simulink model "UseSimDynamicsData"  (R2018b)
settings: configuration reference "RPi_DynamicsRate" (kept outside this file)
values from neighbouring files (symbols this model uses):
  rangeSensorAngBody = [0; 90*dtr; 180*dtr; 270*dtr]    [loadSensorData.m]
  rangeSensorFOV = [0*dtr; 0*dtr; 0*dtr; 0*dtr]    [loadSensorData.m]
  wallBounds = [wallA; wallB; wallC; wallD]    [loadSensorData.m]
undefined symbols (not defined in the file or in its folder): rangeSensorLocBody
settings Model: Creator=barthal  LastModifiedBy=barthal
settings ConfigSetRef: SourceLocation=Base Workspace

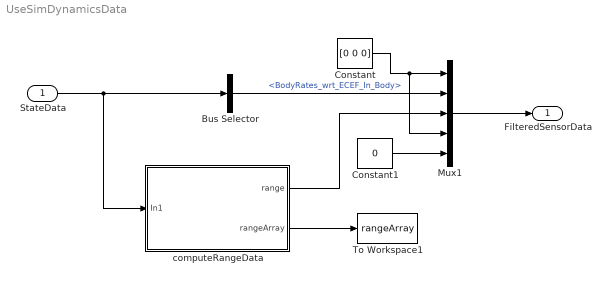
== system UseSimDynamicsData ==
  StateData : Inport  OutDataTypeStr=Bus: FullStateBus
  Bus Selector : BusSelector  OutputSignals=RotState_Body_ECEF.BodyRates_wrt_ECEF_In_Body
  Constant : Constant  Value=[0 0 0]
  Constant1 : Constant  Value=0
  Mux1 : Mux  Inputs=5
  To Workspace1 : ToWorkspace  VariableName=rangeArray  SaveFormat=Timeseries  SampleTime=-1
  computeRangeData : Subsystem
  FilteredSensorData : Outport
  wires:
  StateData/1 -> Bus Selector/1, computeRangeData/1(In1)
  Constant/1 -> Mux1/4, Mux1/1
  Mux1/1 -> FilteredSensorData/1
  computeRangeData/1(range) -> Mux1/3
  computeRangeData/2(rangeArray) -> To Workspace1/1
  Bus Selector/1 -> Mux1/2  "<BodyRates_wrt_ECEF_In_Body>"
  Constant1/1 -> Mux1/5

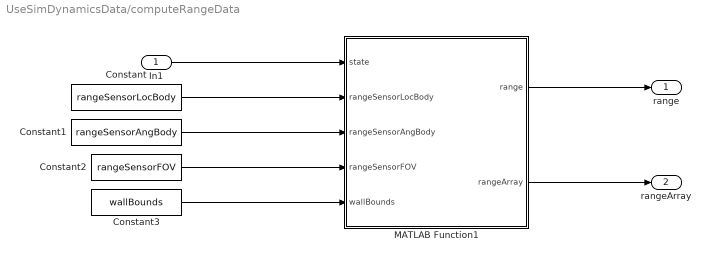
== system UseSimDynamicsData/computeRangeData ==
  In1 : Inport
  Constant : Constant  Value=rangeSensorLocBody
  Constant1 : Constant  Value=rangeSensorAngBody
  Constant2 : Constant  Value=rangeSensorFOV
  Constant3 : Constant  Value=wallBounds
  MATLAB Function1 : MATLAB Function  TreatAsAtomicUnit=on
  range : Outport
  rangeArray : Outport  Port=2
  wires:
  In1/1 -> MATLAB Function1/1(state)
  Constant/1 -> MATLAB Function1/2(rangeSensorLocBody)
  Constant1/1 -> MATLAB Function1/3(rangeSensorAngBody)
  Constant2/1 -> MATLAB Function1/4(rangeSensorFOV)
  MATLAB Function1/1(range) -> range/1
  Constant3/1 -> MATLAB Function1/5(wallBounds)
  MATLAB Function1/2(rangeArray) -> rangeArray/1

== matlab function UseSimDynamicsData/computeRangeData/MATLAB Function1 ==
  data: range output; state input; rangeSensorLocBody input; rangeSensorAngBody input; rangeSensorFOV input; wallBounds input; rangeArray output
function [range,rangeArray] = callsenseWalls(state,rangeSensorLocBody,rangeSensorAngBody,rangeSensorFOV,wallBounds)

[range,rangeArray] = senseWalls(state,rangeSensorLocBody,rangeSensorAngBody,rangeSensorFOV,wallBounds);
